simulink model "Modelo_Nao_Linear_Fase_2_Grupo_10"  (R2016a)
settings: Solver=VariableStepAuto  SolverMode=SingleTasking  StartTime=0.0  StopTime=20  RelTol=1e-3
values from neighbouring files (symbols this model uses):
  A_g = [0 0;1 0]    [Drone_Fase_2.m]
  A_lp = [0  0 0 0; 1 0 0 0; 0 -g 0 0; 0 0 1 0]    [Drone_Fase_2.m]
  A_lr = [0  0 0 0; 1 0 0 0; 0 g 0 0; 0 0 1 0]    [Drone_Fase_2.m]
  A_v = [0 0;1 0]    [Drone_Fase_2.m]
  act2motor_I = K_Omega*inv(act2motor)    [Drone_Fase_2.m]
  B_g = [b_r;0]    [Drone_Fase_2.m]
  B_lp = [b_q;0;0;0]    [Drone_Fase_2.m]
  B_lr = [b_p;0;0;0]    [Drone_Fase_2.m]
  B_v = [-b_z ;0]    [Drone_Fase_2.m]
  C_g = [0  1]    [Drone_Fase_2.m]
  C_lp = [0 1 0 0; 0 0 0 1]    [Drone_Fase_2.m]
  C_lr = [0 1 0 0; 0 0 0 1]    [Drone_Fase_2.m]
  C_v = [0 1]    [Drone_Fase_2.m]
  K_Omega = 3.8013e-4    (= 0.00038013)    [Drone_Fase_2.m]
  K_Q = 1.1393e-10    [Drone_Fase_2.m]
  K_T = 4.72e-8    (= 4.72e-08)    [Drone_Fase_2.m]
  L = 0.0624    [Drone_Fase_2.m]
  m = 0.063    [Drone_Fase_2.m]
  Omega_0 = sqrt((m*g/4)/K_T)    [Drone_Fase_2.m]
  var_omegax = 4.9424*10^(-7)    (= 4.9424e-07)    [Drone_Fase_2.m]
  var_omegay = 5.2748*10^(-7)    (= 5.2748e-07)    [Drone_Fase_2.m]
  var_omegaz = 4.2642*10^(-7)    (= 4.2642e-07)    [Drone_Fase_2.m]
  var_pitch = 2.6060*10^(-4)    (= 0.0002606)    [Drone_Fase_2.m]
  var_px = 7.3221*10^(-4)    (= 0.00073221)    [Drone_Fase_2.m]
  var_py = 4.2829*10^(-4)    (= 0.00042829)    [Drone_Fase_2.m]
  var_pz = 1.8000*10^(-4)    (= 0.00018)    [Drone_Fase_2.m]
  var_roll = 3.4817*10^(-4)    (= 0.00034817)    [Drone_Fase_2.m]
  var_yaw = 3.8313*10^(-5)    (= 3.8313e-05)    [Drone_Fase_2.m]
  Wind = 1e-4*[1; 1; 1]    [Drone_Fase_2.m]
undefined symbols (not defined in the file or in its folder): Lk_g, Lk_lp, Lk_lr, Lk_v, sigbuilder_block
libraries: simulink x6
settings Model: Creator=Ricardo Henriques  LastModifiedBy=Catarina
settings DebuggingCC: SFUnexpectedBacktrackingDiag=error  SFNoUnconditionalDefaultTransitionDiag=error
settings GRTTargetCC: TargetLangStandard=C99 (ISO)  GeneratePreprocessorConditionals=Use local settings
settings ConfigComp: CovMetricSettings=dwe  CovHtmlReporting=off  CovSaveCumulativeToWorkspaceVar=off  CovSaveSingleToWorkspaceVar=off  CovExternalEMLEnable=on

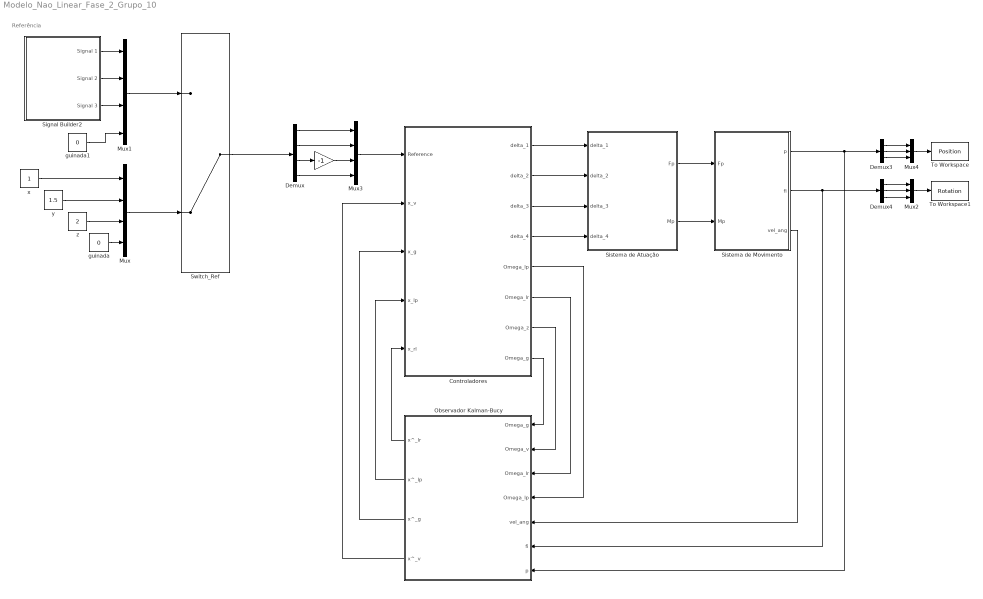
== system Modelo_Nao_Linear_Fase_2_Grupo_10 ==
  note: Referência
  "                " : Gain  Gain=-1
  Controladores : Subsystem
  Demux : Demux
  Demux3 : Demux  Outputs=3
  Demux4 : Demux  Outputs=3
  Mux : Mux
  Mux1 : Mux
  Mux2 : Mux  Inputs=3
  Mux3 : Mux
  Mux4 : Mux  Inputs=3
  Observador Kalman-Bucy : Subsystem
  Signal Builder2 : Subsystem  Tag=STV Subsys  LoadFcn=sigbuilder_block('load');  StartFcn=sigbuilder_block('start');  StopFcn=sigbuilder_block('stop');  ClipboardFcn=sigbuilder_block('clipboard');  mask(Sigbuilder block){}
      mask help: Simulink:masks:SigbuilderBlock_MD
      mask init:
      | if ~strcmp(get_param(bdroot(gcbh),'SimulationStatus'),'stopped') tuvar = sigbuilder_block('maskInit'); end
      settings: CopyFcn=sigbuilder_block('copy');  DeleteFcn=sigbuilder_block('delete');  ModelCloseFcn=sigbuilder_block('modelClose');  PreSaveFcn=sigbuilder_block('preSave');  PauseFcn=sigbuilder_block('pause');  ContinueFcn=sigbuilder_block('continue');  NameChangeFcn=sigbuilder_block('namechange');  OpenFcn=sigbuilder_block('open',[208.2 56.4 858.6 509.4 ]);  CloseFcn=sigbuilder_block('close');
      mask Display: plot(0, 0, 100, 100,[2, 2, 32, 32, 2], [68, 8, 8, 68, 68],[32, 2], [38, 38], [32, 19, 2],[53, 60, 44], [32, 17, 17, 2],[16, 16, 31, 31]);txt = getActiveGroup(gcbh);text(2, 100, txt,'verticalAlignment', 'top');
  Sistema de Atuação : Subsystem
  Sistema de Movimento : Subsystem
  Switch_Ref : ManualSwitch  CurrentSetting=0
  To Workspace : ToWorkspace  VariableName=Position  SaveFormat=Timeseries  SampleTime=1/30
  To Workspace1 : ToWorkspace  VariableName=Rotation  SaveFormat=Timeseries  SampleTime=1/30
  guinada : Constant  Value=0
  guinada1 : Constant  Value=0
  x : Constant
  y : Constant  Value=1.5
  z : Constant  Value=2
  wires:
  Mux/1 -> Switch_Ref/2
  Mux1/1 -> Switch_Ref/1
  Demux4/1 -> Mux2/1
  Demux4/2 -> Mux2/2
  Demux4/3 -> Mux2/3
  Mux2/1 -> To Workspace1/1
  Demux3/1 -> Mux4/1
  Demux3/2 -> Mux4/2
  Demux3/3 -> Mux4/3
  Mux4/1 -> To Workspace/1
  x/1 -> Mux/1
  y/1 -> Mux/2
  guinada/1 -> Mux/4
  z/1 -> Mux/3
  Controladores/7(Omega_z) -> Observador Kalman-Bucy/2(Omega_v)
  Controladores/5(Omega_lp) -> Observador Kalman-Bucy/4(Omega_lp)
  Sistema de Movimento/1(p) -> Demux3/1, Observador Kalman-Bucy/7(p)
  Observador Kalman-Bucy/1(x^_lr) -> Controladores/5(x_rl)
  Observador Kalman-Bucy/2(x^_lp) -> Controladores/4(x_lp)
  Observador Kalman-Bucy/4(x^_v) -> Controladores/2(x_v)
  Controladores/1(delta_1) -> Sistema de Atuação/1(delta_1)
  Controladores/2(delta_2) -> Sistema de Atuação/2(delta_2)
  Controladores/4(delta_4) -> Sistema de Atuação/4(delta_4)
  Sistema de Atuação/2("Mp ") -> Sistema de Movimento/2("Mp ")
  Sistema de Atuação/1(Fp) -> Sistema de Movimento/1(Fp)
  Sistema de Movimento/3(vel_ang) -> Observador Kalman-Bucy/5("vel_ang ")
  guinada1/1 -> Mux1/4
  Observador Kalman-Bucy/3(x^_g) -> Controladores/3(x_g)
  Controladores/6(Omega_lr) -> Observador Kalman-Bucy/3(Omega_lr)
  Controladores/8(Omega_g) -> Observador Kalman-Bucy/1(Omega_g)
  Sistema de Movimento/2(fi) -> Demux4/1, Observador Kalman-Bucy/6("fi ")
  Signal Builder2/1(Signal 1) -> Mux1/1
  Signal Builder2/2(Signal 2) -> Mux1/2
  Signal Builder2/3(Signal 3) -> Mux1/3
  Switch_Ref/1 -> Demux/1
  Demux/3 -> "                "/1
  "                "/1 -> Mux3/3
  Demux/4 -> Mux3/4
  Demux/2 -> Mux3/2
  Demux/1 -> Mux3/1
  Mux3/1 -> Controladores/1(Reference)
  Controladores/3(delta_3) -> Sistema de Atuação/3(delta_3)

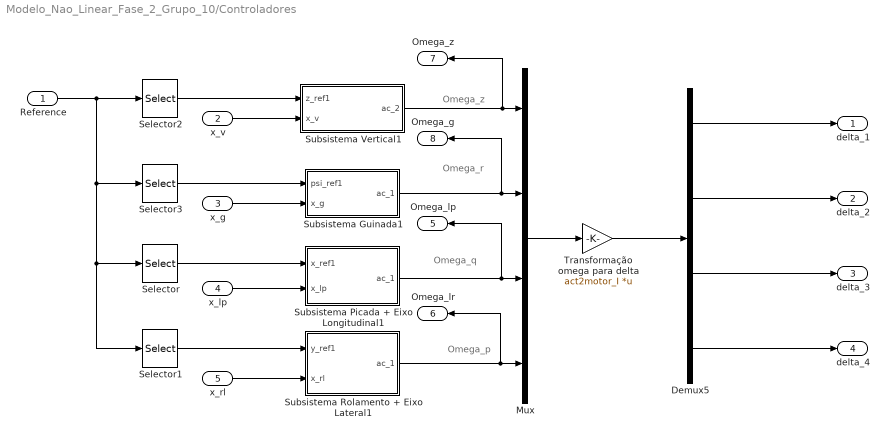
== system Modelo_Nao_Linear_Fase_2_Grupo_10/Controladores ==
  note: Omega_z
  note: Omega_r
  note: Omega_q
  note: Omega_p
  Reference : Inport
  x_v : Inport  Port=2
  x_g : Inport  Port=3
  x_lp : Inport  Port=4
  x_rl : Inport  Port=5
  Demux5 : Demux
  Mux : Mux
  Selector : Selector  InputPortWidth=4  IndexOptions=Index vector (dialog)  Indices=[1]  OutputSizes=1
  Selector1 : Selector  InputPortWidth=4  IndexOptions=Index vector (dialog)  Indices=[2]  OutputSizes=1
  Selector2 : Selector  InputPortWidth=4  IndexOptions=Index vector (dialog)  Indices=[3]  OutputSizes=1
  Selector3 : Selector  InputPortWidth=4  IndexOptions=Index vector (dialog)  Indices=[4]  OutputSizes=1
  Subsistema Guinada1 : Subsystem
  Subsistema Picada + Eixo Longitudinal1 : Subsystem
  Subsistema Rolamento + Eixo Lateral1 : Subsystem
  Subsistema Vertical1 : Subsystem
  Transformação omega para delta : Gain  Gain=act2motor_I  Multiplication=Matrix(K*u) (u vector)
  delta_1 : Outport
  delta_2 : Outport  Port=2
  delta_3 : Outport  Port=3
  delta_4 : Outport  Port=4
  Omega_lp : Outport  Port=5
  Omega_lr : Outport  Port=6
  Omega_z : Outport  Port=7
  Omega_g : Outport  Port=8
  wires:
  Demux5/1 -> delta_1/1
  Demux5/2 -> delta_2/1
  Demux5/3 -> delta_3/1
  Demux5/4 -> delta_4/1
  Subsistema Vertical1/1(ac_2) -> Omega_z/1, Mux/1
  Mux/1 -> Transformação omega para delta/1
  Transformação omega para delta/1 -> Demux5/1
  Subsistema Guinada1/1(ac_1) -> Mux/2, Omega_g/1
  Subsistema Picada + Eixo Longitudinal1/1(ac_1) -> Omega_lp/1, Mux/3
  Subsistema Rolamento + Eixo Lateral1/1(ac_1) -> Mux/4, Omega_lr/1
  x_v/1 -> Subsistema Vertical1/2(x_v)
  x_g/1 -> Subsistema Guinada1/2(x_g)
  x_lp/1 -> Subsistema Picada + Eixo Longitudinal1/2(x_lp)
  x_rl/1 -> Subsistema Rolamento + Eixo Lateral1/2("x_rl ")
  Selector2/1 -> Subsistema Vertical1/1(z_ref1)
  Selector3/1 -> Subsistema Guinada1/1(psi_ref1)
  Selector/1 -> Subsistema Picada + Eixo Longitudinal1/1(x_ref1)
  Selector1/1 -> Subsistema Rolamento + Eixo Lateral1/1(y_ref1)
  Reference/1 -> Selector1/1, Selector/1, Selector3/1, Selector2/1

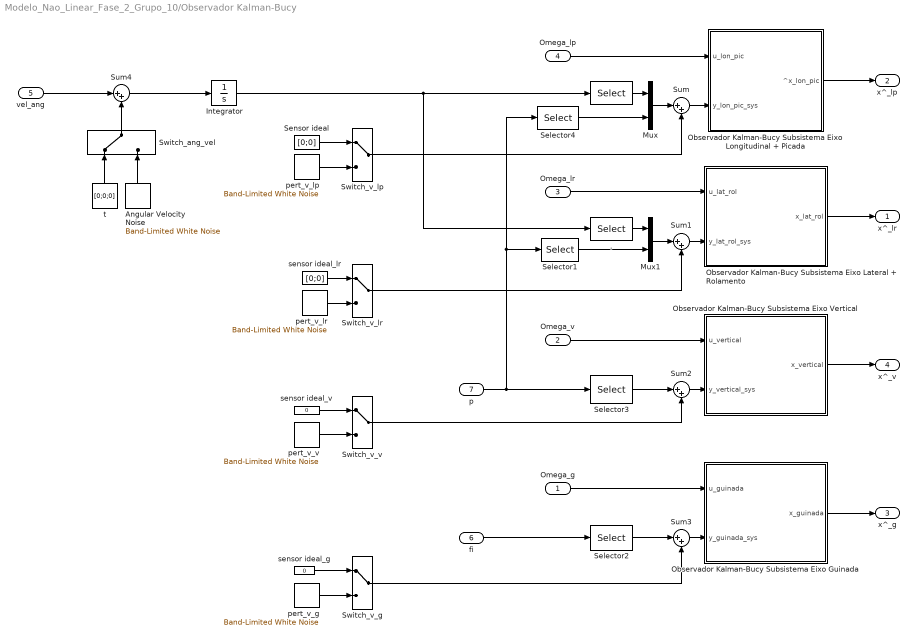
== system Modelo_Nao_Linear_Fase_2_Grupo_10/Observador Kalman-Bucy ==
  Omega_g : Inport
  Omega_v : Inport  Port=2
  Omega_lr : Inport  Port=3
  Omega_lp : Inport  Port=4
  "vel_ang " : Inport  Port=5
  "fi " : Inport  Port=6
  p : Inport  Port=7
  "  " : Selector  InputPortWidth=3  IndexOptions=Index vector (dialog)  Indices=[2]  OutputSizes=1
  "  t" : Constant  Value=[0;0;0]  VectorParams1D=off
  . : Selector  InputPortWidth=3  IndexOptions=Index vector (dialog)  Indices=[1]  OutputSizes=1
  Angular Velocity Noise : simulink/Sources/Band-Limited White Noise  Cov=[var_omegax*0.005; var_omegay*0.005; var_omegaz*0.005]  Ts=0.005  seed=[23341]
  Integrator : Integrator
  Mux : Mux  Inputs=2
  Mux1 : Mux  Inputs=2
  Observador Kalman-Bucy Subsistema Eixo Guinada : Subsystem
  Observador Kalman-Bucy Subsistema Eixo Lateral + Rolamento : Subsystem
  Observador Kalman-Bucy Subsistema Eixo Longitudinal + Picada : Subsystem
  Observador Kalman-Bucy Subsistema Eixo Vertical : Subsystem
  Selector1 : Selector  InputPortWidth=3  IndexOptions=Index vector (dialog)  Indices=[2]  OutputSizes=1
  Selector2 : Selector  InputPortWidth=3  IndexOptions=Index vector (dialog)  Indices=[3]  OutputSizes=1
  Selector3 : Selector  InputPortWidth=3  IndexOptions=Index vector (dialog)  Indices=[3]  OutputSizes=1
  Selector4 : Selector  InputPortWidth=3  IndexOptions=Index vector (dialog)  Indices=[1]  OutputSizes=1
  Sensor ideal : Constant  Value=[0;0]  VectorParams1D=off
  Sum{,1..4} (5 alike) : Sum  Inputs=|++
  Switch_ang_vel : ManualSwitch
  Switch_v_g : ManualSwitch
  Switch_v_lp : ManualSwitch
  Switch_v_lr : ManualSwitch
  Switch_v_v : ManualSwitch
  pert_v_g : simulink/Sources/Band-Limited White Noise  Cov=var_yaw*0.005  Ts=0.005  seed=[23341]
  pert_v_lp : simulink/Sources/Band-Limited White Noise  Cov=[var_pitch*0.005; var_px*0.005]  Ts=0.005  seed=[23341]  VectorParams1D=off
  pert_v_lr : simulink/Sources/Band-Limited White Noise  Cov=[var_roll*0.005; var_py*0.005]  Ts=0.005  seed=[23341]  VectorParams1D=off
  pert_v_v : simulink/Sources/Band-Limited White Noise  Cov=var_pz*0.005  Ts=0.005  seed=[23341]  VectorParams1D=off
  sensor ideal_g : Constant  Value=0  VectorParams1D=off
  sensor ideal_lr : Constant  Value=[0;0]  VectorParams1D=off
  sensor ideal_v : Constant  Value=0  VectorParams1D=off
  x^_lr : Outport
  x^_lp : Outport  Port=2
  x^_g : Outport  Port=3
  x^_v : Outport  Port=4
  wires:
  Omega_v/1 -> Observador Kalman-Bucy Subsistema Eixo Vertical/1(u_vertical)
  Omega_lr/1 -> Observador Kalman-Bucy Subsistema Eixo Lateral + Rolamento/1(u_lat_rol)
  Omega_lp/1 -> Observador Kalman-Bucy Subsistema Eixo Longitudinal + Picada/1(u_lon_pic)
  Omega_g/1 -> Observador Kalman-Bucy Subsistema Eixo Guinada/1(u_guinada)
  Observador Kalman-Bucy Subsistema Eixo Longitudinal + Picada/1(^x_lon_pic) -> x^_lp/1
  Observador Kalman-Bucy Subsistema Eixo Lateral + Rolamento/1(x_lat_rol) -> x^_lr/1
  Observador Kalman-Bucy Subsistema Eixo Vertical/1(x_vertical) -> x^_v/1
  Observador Kalman-Bucy Subsistema Eixo Guinada/1(x_guinada) -> x^_g/1
  pert_v_lp/1 -> Switch_v_lp/2
  Sensor ideal/1 -> Switch_v_lp/1
  Switch_v_lp/1 -> Sum/2
  Mux/1 -> Sum/1
  Sum/1 -> Observador Kalman-Bucy Subsistema Eixo Longitudinal + Picada/2("y_lon_pic_sys ")
  Mux1/1 -> Sum1/1
  Sum1/1 -> Observador Kalman-Bucy Subsistema Eixo Lateral + Rolamento/2("y_lat_rol_sys ")
  sensor ideal_lr/1 -> Switch_v_lr/1
  pert_v_lr/1 -> Switch_v_lr/2
  Switch_v_lr/1 -> Sum1/2
  sensor ideal_v/1 -> Switch_v_v/1
  pert_v_v/1 -> Switch_v_v/2
  Switch_v_v/1 -> Sum2/2
  Sum2/1 -> Observador Kalman-Bucy Subsistema Eixo Vertical/2("y_vertical_sys ")
  sensor ideal_g/1 -> Switch_v_g/1
  Switch_v_g/1 -> Sum3/2
  pert_v_g/1 -> Switch_v_g/2
  Sum3/1 -> Observador Kalman-Bucy Subsistema Eixo Guinada/2("y_guinada_sys ")
  ./1 -> Mux1/1
  Selector1/1 -> Mux1/2
  "  "/1 -> Mux/1
  Selector4/1 -> Mux/2
  p/1 -> Selector4/1, Selector1/1, Selector3/1
  Selector2/1 -> Sum3/1
  Selector3/1 -> Sum2/1
  Switch_ang_vel/1 -> Sum4/2
  "vel_ang "/1 -> Sum4/1
  Sum4/1 -> Integrator/1
  "  t"/1 -> Switch_ang_vel/1
  Angular Velocity Noise/1 -> Switch_ang_vel/2
  Integrator/1 -> "  "/1, ./1
  "fi "/1 -> Selector2/1

== system Modelo_Nao_Linear_Fase_2_Grupo_10/Signal Builder2 ==
  Demux : Demux  Tag=STV Demux  Outputs=3
  FromWs : FromWorkspace  Tag=STV FromWs  VariableName=tuvar  SampleTime=0
      SigBuilderData=|
      | common.afterFinalStr = 'Extrapolate'
      | common.sampleTime = 0
      | dataSet.timeRange = [0 60]
      | dataSet.name = 'Group 1'
      | sbobj.Groups.Name = 'Group 1'
      | sbobj.Groups.Signals(1).Name = 'Signal 1'
      | sbobj.Groups.Signals(1).XData = [0 1 2 3 4 5 6 7 8 9 10 10 11 12 13 14 15 16 17 18 19 20 21 22 23 24 25 26 27 28 29 30 31 32 33 34 35 36 37 38 39 40 41 42 43 44 45 46 47 48 49 50 51 52 53 54 55 56 57 58 59 60]
      | sbobj.Groups.Signals(1).YData = [0 0 0 0 0 0 0 0 2 2 1.98 2 2 2 2 2 2 2 2 2 2 -2 -2 -2 -2 -2 -2 -2 -2 2 2 2 2 2 2 2 2 2 2 2 2 -2 -2 -2 -2 -2 -2 -2 -2 -2 -2 2 2 2 2 2 2 2 0 0 0 0]
      | sbobj.Groups.Signals(2).Name = 'Signal 2'
      | sbobj.Groups.Signals(2).XData = [0 1 2 3 4 4 5 6 7 8 9 10 11 12 13 14 15 16 17 18 19 20 21 22 23 24 25 26 27 28 29 30 31 32 33 34 35 36 37 38 39 40 41 42 43 44 45 46 47 48 49 50 51 52 53 54 55 56 57 58 59 60]
      | sbobj.Groups.Signals(2).YData = [0 2 2 2 1.98 2 2 2 2 -2 -2 -2 -2 -2 -2 -2 -2 -2 -2 -2 -2 2 2 2 2 2 2 2 2 2 2 2 2 -2 -2 -2 -2 -2 -2 -2 -2 -2 -2 -2 -2 2 2 2 2 2 2 2 2 2 2 2 2 -2 -2 -1.95 -2 -2]
      | sbobj.Groups.Signals(3).Name = 'Signal 3'
      | sbobj.Groups.Signals(3).XData = [0 24 36 55 60]
      | sbobj.Groups.Signals(3).YData = [0 1 1 0 0]
      | sbobj.Groups.TimeRange = [0 60]
  Signal 1 : Outport  Tag=STV Outport
  Signal 2 : Outport  Tag=STV Outport  Port=2
  Signal 3 : Outport  Tag=STV Outport  Port=3
  wires:
  FromWs/1 -> Demux/1
  Demux/1 -> Signal 1/1
  Demux/2 -> Signal 2/1
  Demux/3 -> Signal 3/1

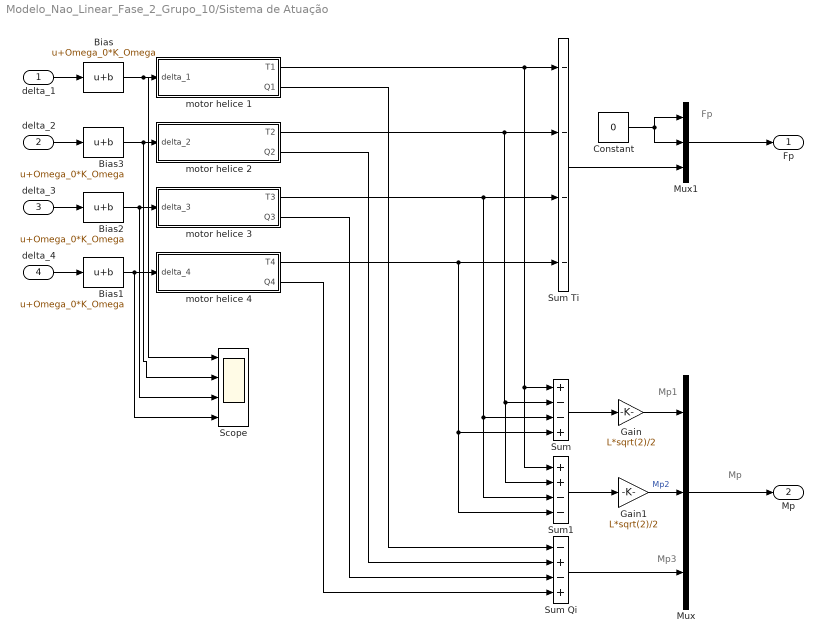
== system Modelo_Nao_Linear_Fase_2_Grupo_10/Sistema de Atuação ==
  note: Fp
  note: Mp
  note: Mp1
  note: Mp3
  delta_1 : Inport
  delta_2 : Inport  Port=2
  delta_3 : Inport  Port=3
  delta_4 : Inport  Port=4
  Bias{,1..3} (4 alike) : Bias  Bias=Omega_0*K_Omega
  Constant : Constant  Value=0
  Gain : Gain  Gain=L*sqrt(2)/2
  Gain1 : Gain  Gain=L*sqrt(2)/2
  Mux : Mux  Inputs=3
  Mux1 : Mux  Inputs=3
  Scope : Scope  NumInputPorts=4
  Sum : Sum  Inputs=+--+
  Sum Qi : Sum  Inputs=-+-+
  Sum Ti : Sum  Inputs=----
  Sum1 : Sum  Inputs=++--
  motor helice 1 : Subsystem
  motor helice 2 : Subsystem
  motor helice 3 : Subsystem
  motor helice 4 : Subsystem
  Fp : Outport
  "Mp " : Outport  Port=2
  wires:
  Sum/1 -> Gain/1
  Mux/1 -> "Mp "/1
  Gain1/1 -> Mux/2  "Mp2"
  Sum1/1 -> Gain1/1
  Sum Ti/1 -> Mux1/3
  Constant/1 -> Mux1/2, Mux1/1
  Mux1/1 -> Fp/1
  Gain/1 -> Mux/1
  Sum Qi/1 -> Mux/3
  motor helice 1/1(T1) -> Sum1/1, Sum/1, Sum Ti/1
  motor helice 2/1(T2) -> Sum1/2, Sum/2, Sum Ti/2
  motor helice 3/1(T3) -> Sum1/3, Sum/3, Sum Ti/3
  motor helice 4/1(T4) -> Sum/4, Sum1/4, Sum Ti/4
  motor helice 1/2(Q1) -> Sum Qi/1
  motor helice 2/2(Q2) -> Sum Qi/2
  motor helice 3/2(Q3) -> Sum Qi/3
  motor helice 4/2(Q4) -> Sum Qi/4
  delta_1/1 -> Bias/1
  delta_4/1 -> Bias1/1
  delta_3/1 -> Bias2/1
  delta_2/1 -> Bias3/1
  Bias1/1 -> Scope/4, motor helice 4/1(delta_4)
  Bias3/1 -> Scope/2, motor helice 2/1(delta_2)
  Bias2/1 -> Scope/3, motor helice 3/1(delta_3)
  Bias/1 -> Scope/1, motor helice 1/1(delta_1)

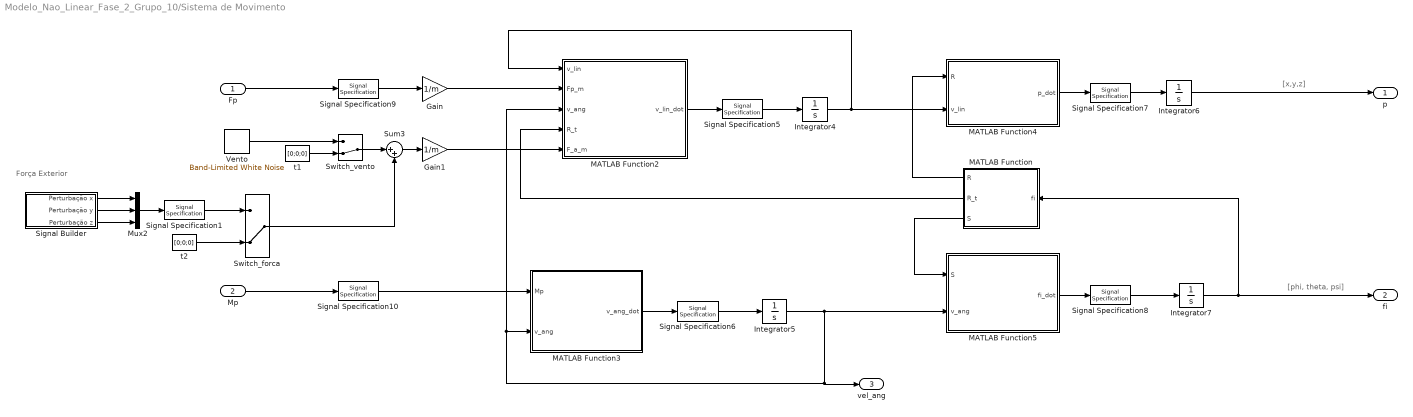
== system Modelo_Nao_Linear_Fase_2_Grupo_10/Sistema de Movimento ==
  note: Força Exterior
  note: [phi, theta, psi]
  note: [x,y,z]
  Fp : Inport
  "Mp " : Inport  Port=2
  "  t1" : Constant  Value=[0;0;0]  VectorParams1D=off
  "  t2" : Constant  Value=[0;0;0]  VectorParams1D=off
  Gain : Gain  Gain=1/m
  Gain1 : Gain  Gain=1/m
  Integrator4 : Integrator
  Integrator5 : Integrator
  Integrator6 : Integrator  InitialCondition=[0;0;0]
  Integrator7 : Integrator  InitialCondition=[0;0;0]
  MATLAB Function : MATLAB Function  TreatAsAtomicUnit=on
  MATLAB Function2 : MATLAB Function  TreatAsAtomicUnit=on
  MATLAB Function3 : MATLAB Function  TreatAsAtomicUnit=on
  MATLAB Function4 : MATLAB Function  TreatAsAtomicUnit=on
  MATLAB Function5 : MATLAB Function  TreatAsAtomicUnit=on
  Mux2 : Mux  Inputs=3
  Signal Builder : Subsystem  Tag=STV Subsys  LoadFcn=sigbuilder_block('load');  StartFcn=sigbuilder_block('start');  StopFcn=sigbuilder_block('stop');  ClipboardFcn=sigbuilder_block('clipboard');  mask(Sigbuilder block){}
      mask help: Simulink:masks:SigbuilderBlock_MD
      mask init:
      | if ~strcmp(get_param(bdroot(gcbh),'SimulationStatus'),'stopped') tuvar = sigbuilder_block('maskInit'); end
      settings: CopyFcn=sigbuilder_block('copy');  DeleteFcn=sigbuilder_block('delete');  ModelCloseFcn=sigbuilder_block('modelClose');  PreSaveFcn=sigbuilder_block('preSave');  PauseFcn=sigbuilder_block('pause');  ContinueFcn=sigbuilder_block('continue');  NameChangeFcn=sigbuilder_block('namechange');  OpenFcn=sigbuilder_block('open',[5.4 30 1141.2 522.6 ]);  CloseFcn=sigbuilder_block('close');
      mask Display: plot(0, 0, 100, 100,[2, 2, 32, 32, 2], [68, 8, 8, 68, 68],[32, 2], [38, 38], [32, 19, 2],[53, 60, 44], [32, 17, 17, 2],[16, 16, 31, 31]);txt = getActiveGroup(gcbh);text(2, 100, txt,'verticalAlignment', 'top');
  Signal Specification{1,5..10} (7 alike) : SignalSpecification  Dimensions=[3 1]
  Sum3 : Sum  Inputs=|++
  Switch_forca : ManualSwitch  CurrentSetting=0
  Switch_vento : ManualSwitch  CurrentSetting=0
  "Vento " : simulink/Sources/Band-Limited White Noise  Cov=Wind*0.005  Ts=0.005  seed=[23341]  VectorParams1D=off
  p : Outport
  fi : Outport  Port=2
  vel_ang : Outport  Port=3
  wires:
  Fp/1 -> Signal Specification9/1
  Signal Specification5/1 -> Integrator4/1
  MATLAB Function2/1(v_lin_dot) -> Signal Specification5/1
  MATLAB Function3/1(v_ang_dot) -> Signal Specification6/1
  MATLAB Function4/1(p_dot) -> Signal Specification7/1
  MATLAB Function5/1(fi_dot) -> Signal Specification8/1
  Signal Specification9/1 -> Gain/1
  "Mp "/1 -> Signal Specification10/1
  Signal Specification10/1 -> MATLAB Function3/1(Mp)
  Gain/1 -> MATLAB Function2/2(Fp_m)
  MATLAB Function/2(R_t) -> MATLAB Function2/4(R_t)
  MATLAB Function/3(S) -> MATLAB Function5/1(S)
  MATLAB Function/1(R) -> MATLAB Function4/1(R)
  Integrator4/1 -> MATLAB Function4/2(v_lin), MATLAB Function2/1(v_lin)
  Gain1/1 -> MATLAB Function2/5(F_a_m)
  Signal Builder/1(Perturbação x) -> Mux2/1
  Signal Builder/2(Perturbação y) -> Mux2/2
  Signal Builder/3(Perturbação z) -> Mux2/3
  Mux2/1 -> Signal Specification1/1
  Signal Specification6/1 -> Integrator5/1
  Integrator6/1 -> p/1
  Signal Specification7/1 -> Integrator6/1
  Integrator7/1 -> fi/1, MATLAB Function/1(fi)
  Signal Specification8/1 -> Integrator7/1
  "  t1"/1 -> Switch_vento/2
  Signal Specification1/1 -> Switch_forca/1
  "  t2"/1 -> Switch_forca/2
  Switch_forca/1 -> Sum3/2
  Integrator5/1 -> vel_ang/1, MATLAB Function2/3(v_ang), MATLAB Function3/2(v_ang), MATLAB Function5/2(v_ang)
  "Vento "/1 -> Switch_vento/1
  Sum3/1 -> Gain1/1
  Switch_vento/1 -> Sum3/1

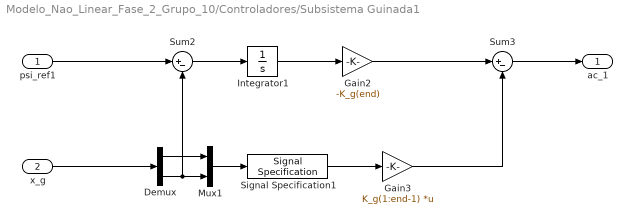
== system Modelo_Nao_Linear_Fase_2_Grupo_10/Controladores/Subsistema Guinada1 ==
  psi_ref1 : Inport
  x_g : Inport  Port=2
  Demux : Demux  Outputs=2
  Gain2 : Gain  Gain=-K_g(end)
  Gain3 : Gain  Gain=K_g(1:end-1)  Multiplication=Matrix(K*u) (u vector)
  Integrator1 : Integrator
  Mux1 : Mux  Inputs=2
  Signal Specification1 : SignalSpecification  Dimensions=[2 1]
  Sum2 : Sum  Inputs=|+-
  Sum3 : Sum  Inputs=|+-
  ac_1 : Outport
  wires:
  Gain3/1 -> Sum3/2
  Gain2/1 -> Sum3/1
  Integrator1/1 -> Gain2/1
  Signal Specification1/1 -> Gain3/1
  Mux1/1 -> Signal Specification1/1
  Sum3/1 -> ac_1/1
  psi_ref1/1 -> Sum2/1
  Sum2/1 -> Integrator1/1
  x_g/1 -> Demux/1
  Demux/1 -> Mux1/1
  Demux/2 -> Sum2/2, Mux1/2

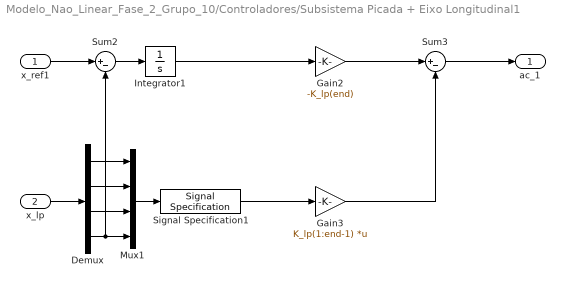
== system Modelo_Nao_Linear_Fase_2_Grupo_10/Controladores/Subsistema Picada + Eixo Longitudinal1 ==
  x_ref1 : Inport
  x_lp : Inport  Port=2
  Demux : Demux
  Gain2 : Gain  Gain=-K_lp(end)
  Gain3 : Gain  Gain=K_lp(1:end-1)  Multiplication=Matrix(K*u) (u vector)
  Integrator1 : Integrator
  Mux1 : Mux
  Signal Specification1 : SignalSpecification  Dimensions=[4 1]
  Sum2 : Sum  Inputs=|+-
  Sum3 : Sum  Inputs=|+-
  ac_1 : Outport
  wires:
  x_ref1/1 -> Sum2/1
  Sum2/1 -> Integrator1/1
  Integrator1/1 -> Gain2/1
  Gain2/1 -> Sum3/1
  Sum3/1 -> ac_1/1
  Gain3/1 -> Sum3/2
  Mux1/1 -> Signal Specification1/1
  Signal Specification1/1 -> Gain3/1
  Demux/1 -> Mux1/1
  Demux/2 -> Mux1/2
  Demux/3 -> Mux1/3
  Demux/4 -> Sum2/2, Mux1/4
  x_lp/1 -> Demux/1

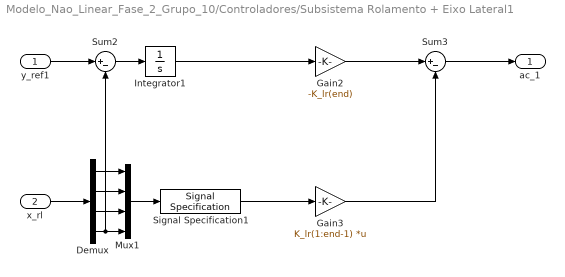
== system Modelo_Nao_Linear_Fase_2_Grupo_10/Controladores/Subsistema Rolamento + Eixo Lateral1 ==
  y_ref1 : Inport
  "x_rl " : Inport  Port=2
  Demux : Demux
  Gain2 : Gain  Gain=-K_lr(end)
  Gain3 : Gain  Gain=K_lr(1:end-1)  Multiplication=Matrix(K*u) (u vector)
  Integrator1 : Integrator
  Mux1 : Mux
  Signal Specification1 : SignalSpecification  Dimensions=[4 1]
  Sum2 : Sum  Inputs=|+-
  Sum3 : Sum  Inputs=|+-
  ac_1 : Outport
  wires:
  y_ref1/1 -> Sum2/1
  Sum2/1 -> Integrator1/1
  Integrator1/1 -> Gain2/1
  Gain2/1 -> Sum3/1
  Sum3/1 -> ac_1/1
  Gain3/1 -> Sum3/2
  Signal Specification1/1 -> Gain3/1
  "x_rl "/1 -> Demux/1
  Demux/1 -> Mux1/1
  Demux/2 -> Mux1/2
  Demux/3 -> Mux1/3
  Demux/4 -> Mux1/4, Sum2/2
  Mux1/1 -> Signal Specification1/1

== system Modelo_Nao_Linear_Fase_2_Grupo_10/Controladores/Subsistema Vertical1 ==
  z_ref1 : Inport
  x_v : Inport  Port=2
  Demux : Demux  Outputs=2
  Gain2 : Gain  Gain=-K_v(end)
  Gain3 : Gain  Gain=K_v(1:end-1)  Multiplication=Matrix(K*u) (u vector)
  Integrator1 : Integrator
  Mux1 : Mux  Inputs=2
  Signal Specification1 : SignalSpecification  Dimensions=[2 1]
  Sum2 : Sum  Inputs=|+-
  Sum3 : Sum  Inputs=|+-
  ac_2 : Outport
  wires:
  z_ref1/1 -> Sum2/1
  Sum2/1 -> Integrator1/1
  Integrator1/1 -> Gain2/1
  Mux1/1 -> Signal Specification1/1
  Gain2/1 -> Sum3/1
  Gain3/1 -> Sum3/2
  Sum3/1 -> ac_2/1
  Signal Specification1/1 -> Gain3/1
  x_v/1 -> Demux/1
  Demux/2 -> Sum2/2, Mux1/2
  Demux/1 -> Mux1/1

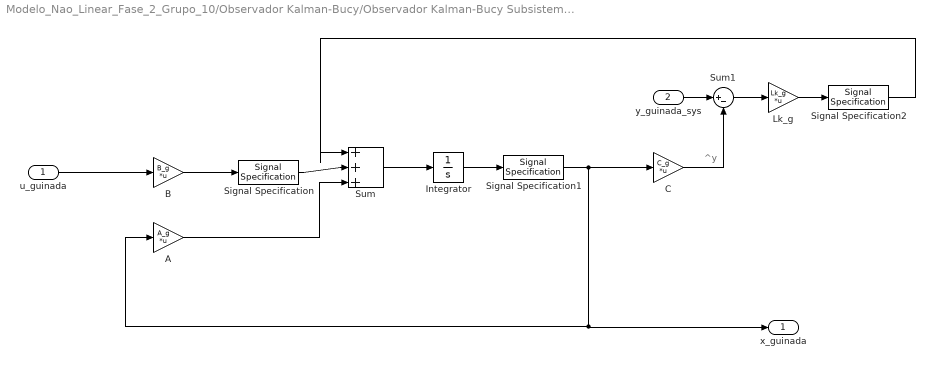
== system Modelo_Nao_Linear_Fase_2_Grupo_10/Observador Kalman-Bucy/Observador Kalman-Bucy Subsistema Eixo Guinada ==
  note: ^y
  u_guinada : Inport
  "y_guinada_sys " : Inport  Port=2
  A : Gain  Gain=A_g  Multiplication=Matrix(K*u)
  B : Gain  Gain=B_g  Multiplication=Matrix(K*u)
  C : Gain  Gain=C_g  Multiplication=Matrix(K*u)
  Integrator : Integrator  InitialCondition=[0;0]
  Lk_g : Gain  Gain=Lk_g  Multiplication=Matrix(K*u) (u vector)
  Signal Specification : SignalSpecification  Dimensions=[2 1]
  Signal Specification1 : SignalSpecification  Dimensions=[2 1]
  Signal Specification2 : SignalSpecification  Dimensions=[2 1]
  Sum : Sum  Inputs=|+++
  Sum1 : Sum  Inputs=|+-
  x_guinada : Outport
  wires:
  B/1 -> Signal Specification/1
  Sum/1 -> Integrator/1
  Integrator/1 -> Signal Specification1/1
  A/1 -> Sum/3
  Signal Specification1/1 -> x_guinada/1, A/1, C/1
  u_guinada/1 -> B/1
  C/1 -> Sum1/2
  Signal Specification/1 -> Sum/2
  "y_guinada_sys "/1 -> Sum1/1
  Sum1/1 -> Lk_g/1
  Lk_g/1 -> Signal Specification2/1
  Signal Specification2/1 -> Sum/1

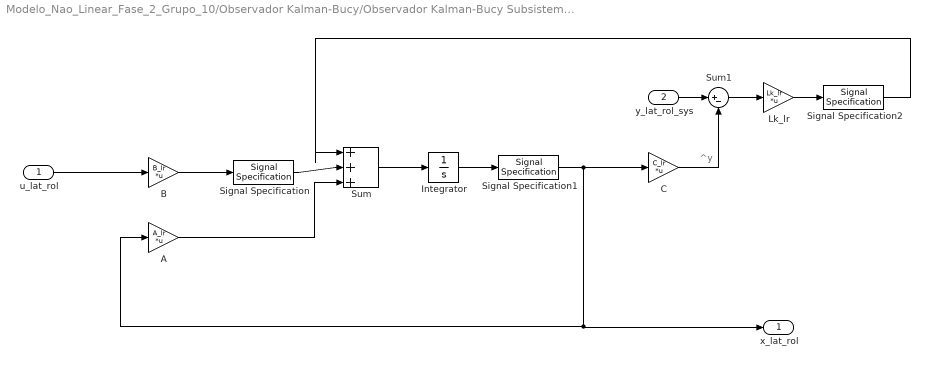
== system Modelo_Nao_Linear_Fase_2_Grupo_10/Observador Kalman-Bucy/Observador Kalman-Bucy Subsistema Eixo Lateral + Rolamento ==
  note: ^y
  u_lat_rol : Inport
  "y_lat_rol_sys " : Inport  Port=2
  A : Gain  Gain=A_lr  Multiplication=Matrix(K*u)
  B : Gain  Gain=B_lr  Multiplication=Matrix(K*u)
  C : Gain  Gain=C_lr  Multiplication=Matrix(K*u)
  Integrator : Integrator  InitialCondition=[0;0;0;0]
  Lk_lr : Gain  Gain=Lk_lr  Multiplication=Matrix(K*u) (u vector)
  Signal Specification : SignalSpecification  Dimensions=[4 1]
  Signal Specification1 : SignalSpecification  Dimensions=[4 1]
  Signal Specification2 : SignalSpecification  Dimensions=[4 1]
  Sum : Sum  Inputs=|+++
  Sum1 : Sum  Inputs=|+-
  x_lat_rol : Outport
  wires:
  B/1 -> Signal Specification/1
  Sum/1 -> Integrator/1
  Integrator/1 -> Signal Specification1/1
  A/1 -> Sum/3
  Signal Specification1/1 -> x_lat_rol/1, A/1, C/1
  u_lat_rol/1 -> B/1
  C/1 -> Sum1/2
  Signal Specification/1 -> Sum/2
  "y_lat_rol_sys "/1 -> Sum1/1
  Sum1/1 -> Lk_lr/1
  Lk_lr/1 -> Signal Specification2/1
  Signal Specification2/1 -> Sum/1

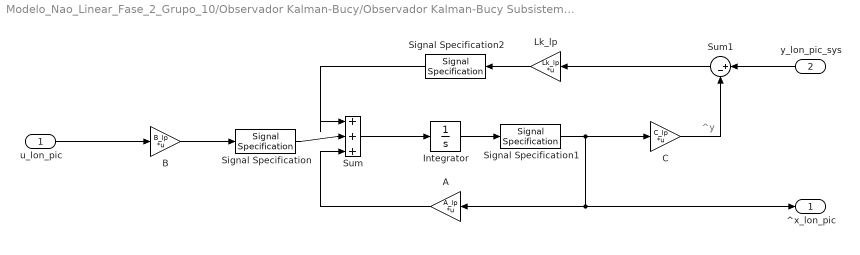
== system Modelo_Nao_Linear_Fase_2_Grupo_10/Observador Kalman-Bucy/Observador Kalman-Bucy Subsistema Eixo Longitudinal + Picada ==
  note: ^y
  u_lon_pic : Inport
  "y_lon_pic_sys " : Inport  Port=2
  A : Gain  Gain=A_lp  Multiplication=Matrix(K*u)
  B : Gain  Gain=B_lp  Multiplication=Matrix(K*u)
  C : Gain  Gain=C_lp  Multiplication=Matrix(K*u)
  Integrator : Integrator  InitialCondition=[0;0;0;0]
  Lk_lp : Gain  Gain=Lk_lp  Multiplication=Matrix(K*u) (u vector)
  Signal Specification : SignalSpecification  Dimensions=[4 1]
  Signal Specification1 : SignalSpecification  Dimensions=[4 1]
  Signal Specification2 : SignalSpecification  Dimensions=[4 1]
  Sum : Sum  Inputs=|+++
  Sum1 : Sum  Inputs=|+-
  ^x_lon_pic : Outport
  wires:
  B/1 -> Signal Specification/1
  Sum/1 -> Integrator/1
  Integrator/1 -> Signal Specification1/1
  A/1 -> Sum/3
  Signal Specification1/1 -> ^x_lon_pic/1, A/1, C/1
  u_lon_pic/1 -> B/1
  C/1 -> Sum1/2
  Signal Specification/1 -> Sum/2
  "y_lon_pic_sys "/1 -> Sum1/1
  Sum1/1 -> Lk_lp/1
  Lk_lp/1 -> Signal Specification2/1
  Signal Specification2/1 -> Sum/1

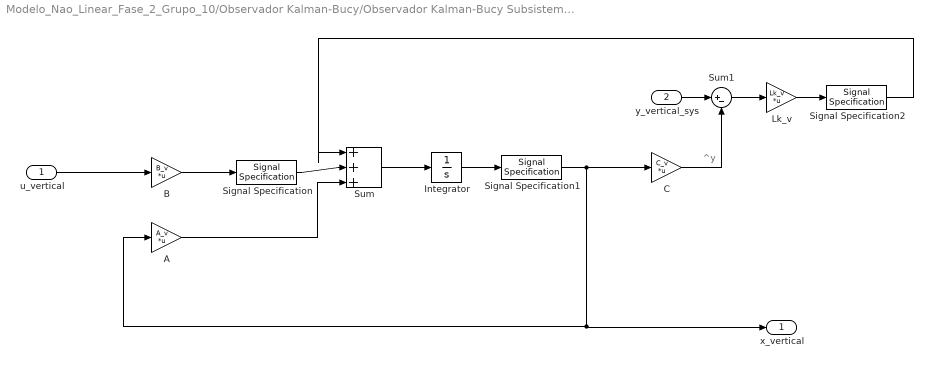
== system Modelo_Nao_Linear_Fase_2_Grupo_10/Observador Kalman-Bucy/Observador Kalman-Bucy Subsistema Eixo Vertical ==
  note: ^y
  u_vertical : Inport
  "y_vertical_sys " : Inport  Port=2
  A : Gain  Gain=A_v  Multiplication=Matrix(K*u)
  B : Gain  Gain=B_v  Multiplication=Matrix(K*u)
  C : Gain  Gain=C_v  Multiplication=Matrix(K*u)
  Integrator : Integrator  InitialCondition=[0;0]
  Lk_v : Gain  Gain=Lk_v  Multiplication=Matrix(K*u) (u vector)
  Signal Specification : SignalSpecification  Dimensions=[2 1]
  Signal Specification1 : SignalSpecification  Dimensions=[2 1]
  Signal Specification2 : SignalSpecification  Dimensions=[2 1]
  Sum : Sum  Inputs=|+++
  Sum1 : Sum  Inputs=|+-
  x_vertical : Outport
  wires:
  B/1 -> Signal Specification/1
  Sum/1 -> Integrator/1
  Integrator/1 -> Signal Specification1/1
  A/1 -> Sum/3
  Signal Specification1/1 -> x_vertical/1, A/1, C/1
  u_vertical/1 -> B/1
  C/1 -> Sum1/2
  Signal Specification/1 -> Sum/2
  "y_vertical_sys "/1 -> Sum1/1
  Sum1/1 -> Lk_v/1
  Lk_v/1 -> Signal Specification2/1
  Signal Specification2/1 -> Sum/1

== system Modelo_Nao_Linear_Fase_2_Grupo_10/Sistema de Atuação/motor helice 1 ==
  note: Q1
  note: T1
  delta_1 : Inport
  Gain6 : Gain  Gain=K_T
  Gain7 : Gain  Gain=K_Q
  Math Function1 : Math  Operator=square  SaturateOnIntegerOverflow=on
  Motor 1 : Gain  Gain=1/K_Omega
  Saturation : Saturate  UpperLimit=1  LowerLimit=0
  T1 : Outport
  Q1 : Outport  Port=2
  wires:
  delta_1/1 -> Saturation/1
  Motor 1/1 -> Math Function1/1
  Math Function1/1 -> Gain7/1, Gain6/1
  Gain6/1 -> T1/1
  Gain7/1 -> Q1/1
  Saturation/1 -> Motor 1/1

== system Modelo_Nao_Linear_Fase_2_Grupo_10/Sistema de Atuação/motor helice 2 ==
  note: T2
  note: Q2
  delta_2 : Inport
  Gain6 : Gain  Gain=K_T
  Gain7 : Gain  Gain=K_Q
  Math Function1 : Math  Operator=square  SaturateOnIntegerOverflow=on
  Motor 2 : Gain  Gain=1/K_Omega
  Saturation : Saturate  UpperLimit=1  LowerLimit=0
  T2 : Outport
  Q2 : Outport  Port=2
  wires:
  Gain7/1 -> Q2/1
  Motor 2/1 -> Math Function1/1
  Math Function1/1 -> Gain7/1, Gain6/1
  Saturation/1 -> Motor 2/1
  delta_2/1 -> Saturation/1
  Gain6/1 -> T2/1

== system Modelo_Nao_Linear_Fase_2_Grupo_10/Sistema de Atuação/motor helice 3 ==
  note: T3
  note: Q3
  delta_3 : Inport
  Gain6 : Gain  Gain=K_T
  Gain7 : Gain  Gain=K_Q
  Math Function1 : Math  Operator=square  SaturateOnIntegerOverflow=on
  Motor 3 : Gain  Gain=1/K_Omega
  Saturation : Saturate  UpperLimit=1  LowerLimit=0
  T3 : Outport
  Q3 : Outport  Port=2
  wires:
  Gain7/1 -> Q3/1
  Motor 3/1 -> Math Function1/1
  Math Function1/1 -> Gain7/1, Gain6/1
  Saturation/1 -> Motor 3/1
  delta_3/1 -> Saturation/1
  Gain6/1 -> T3/1

== system Modelo_Nao_Linear_Fase_2_Grupo_10/Sistema de Atuação/motor helice 4 ==
  note: T4
  note: Q4
  delta_4 : Inport
  Gain6 : Gain  Gain=K_T
  Gain7 : Gain  Gain=K_Q
  Math Function1 : Math  Operator=square  SaturateOnIntegerOverflow=on
  Motor 4 : Gain  Gain=1/K_Omega
  Saturation : Saturate  UpperLimit=1  LowerLimit=0
  T4 : Outport
  Q4 : Outport  Port=2
  wires:
  Gain7/1 -> Q4/1
  Motor 4/1 -> Math Function1/1
  Math Function1/1 -> Gain7/1, Gain6/1
  Saturation/1 -> Motor 4/1
  delta_4/1 -> Saturation/1
  Gain6/1 -> T4/1

== system Modelo_Nao_Linear_Fase_2_Grupo_10/Sistema de Movimento/Signal Builder ==
  Demux : Demux  Tag=STV Demux  Outputs=3
  FromWs : FromWorkspace  Tag=STV FromWs  VariableName=tuvar  SampleTime=0
      SigBuilderData=|
      | common.afterFinalStr = 'Extrapolate'
      | common.sampleTime = 0
      | dataSet.timeRange = [0 60]
      | dataSet.name = 'Group 1'
      | sbobj.Groups.Name = 'Group 1'
      | sbobj.Groups.Signals(1).Name = 'Perturbação x'
      | sbobj.Groups.Signals(1).XData = [0 20.05 20.05 30 30 60]
      | sbobj.Groups.Signals(1).YData = [0 0 0.053 0.0135 0 0]
      | sbobj.Groups.Signals(2).Name = 'Perturbação y'
      | sbobj.Groups.Signals(2).XData = [0 7.65 7.65 16.35 16.35 60]
      | sbobj.Groups.Signals(2).YData = [0 0.0005 0.0395 0.039 0 0]
      | sbobj.Groups.Signals(3).Name = 'Perturbação z'
      | sbobj.Groups.Signals(3).XData = [0 38.6 38.6 45.1 53.75 53.75 60]
      | sbobj.Groups.Signals(3).YData = [0 0 0.029 0.07 0.01 0.001 0]
      | sbobj.Groups.TimeRange = [0 60]
  Perturbação x : Outport  Tag=STV Outport
  Perturbação y : Outport  Tag=STV Outport  Port=2
  Perturbação z : Outport  Tag=STV Outport  Port=3
  wires:
  Demux/1 -> Perturbação x/1
  FromWs/1 -> Demux/1
  Demux/2 -> Perturbação y/1
  Demux/3 -> Perturbação z/1

== matlab function Modelo_Nao_Linear_Fase_2_Grupo_10/Sistema de Movimento/MATLAB Function ==
  data: R output; R_t output; fi input; S output
function [R,R_t,S] = matrizes_R_S(fi)

s_x = sin(fi(1));
s_y = sin(fi(2));
s_z = sin(fi(3));

c_x = cos(fi(1));
c_y = cos(fi(2));
c_z = cos(fi(3));

t_x = tan(fi(1));
t_y = tan(fi(2));

S = [1   s_x*t_y   c_x*t_y;
     0   c_x       -s_x;
     0   t_x       c_x/c_y];
 
R = [c_z*c_y     (c_z*s_y*s_x)-(s_z*c_x)  (c_z*s_y*c_x)+(s_z*s_x);
     s_z*c_y     (s_z*s_y*s_x)+(c_z*c_x)  (s_z*s_y*c_x)-(c_z*s_x);
     -s_y         c_y*s_x                  c_y*c_x              ];

R_t = transpose(R);
end

== matlab function Modelo_Nao_Linear_Fase_2_Grupo_10/Sistema de Movimento/MATLAB Function2 ==
  data: v_lin input; Fp_m input; v_ang input; R_t input; v_lin_dot output; F_a_m input
function v_lin_dot = derivada_v_lin(v_lin,Fp_m,v_ang,R_t,F_a_m)
g = 9.81;
v_lin_dot = cross(-v_ang,v_lin) + R_t*[0;0;g] + Fp_m + F_a_m;
end

== matlab function Modelo_Nao_Linear_Fase_2_Grupo_10/Sistema de Movimento/MATLAB Function3 ==
  data: Mp input; v_ang_dot output; v_ang input
function v_ang_dot = derivada_v_ang(Mp,v_ang)

J_x    =    5.8286e-5;                            %Kg.m^2
J_y    =    7.1691e-5;                            %Kg.m^2
J_z    =    1.0e-4;                               %Kg.m^2
J = [J_x   0    0;
       0 J_y    0;
       0   0  J_z];

J_i = inv(J);
v_ang_dot = cross(-J_i*v_ang,J*v_ang) + J_i*Mp;
end

== matlab function Modelo_Nao_Linear_Fase_2_Grupo_10/Sistema de Movimento/MATLAB Function4 ==
  data: R input; p_dot output; v_lin input
function p_dot = derivada_posicao(R,v_lin)
p_dot = R*v_lin;
end

== matlab function Modelo_Nao_Linear_Fase_2_Grupo_10/Sistema de Movimento/MATLAB Function5 ==
  data: S input; fi_dot output; v_ang input
function fi_dot = derivada_posicao_angular(S,v_ang)
fi_dot = S*v_ang;
end
